simulink model "tesd"  (R2012b)
settings: Solver=ode45  StartTime=0.0  StopTime=25000  RelTol=1e-3
undefined symbols (not defined in the file or in its folder): pfb_coeff_gen_calc, sfp
undefined symbols (not defined in the file): SL, transtable
libraries: xbsIndex_r4 x5040, casper_library_misc x112, casper_library_delays x24, xps_library x14, maddogLibrary x4, simulink x2
(part 34 of 49)

== system tesd/FRD1/trIQ/tr/mem ==
  note: Undo data manipulation on way in and redo on way out for simulated data
  note: Undo address
      | manipulation for
      | simulated data
  In1 : Inport
  In2 : Inport  Port=2
  In3 : Inport  Port=3
  Disregard Subsystem : xbsIndex_r4/Disregard Subsystem  Tag=discardX  block_type=disregard
  calc_add : Subsystem  mask{data_width=32, addr_width=10, sample_rate=sample_rate}
      mask prompts: data_width "data width"; addr_width "address width"; sample_rate "sample rate"
  ram : xbsIndex_r4/Single Port RAM  depth=2^addr_width  initVector=init_vals  distributed_mem=Block RAM  write_mode=Read After Write  rst=off  init_reg=0  en=off  latency=1  dbl_ovrd=off  optimize=Area  block_type=spram
  sim_addr : xbsIndex_r4/Gateway In  gui_display_data_type=Fixed-point  arith_type=Unsigned  n_bits=addr_width  bin_pt=0  preci_type=Single  exp_width=8  frac_width=24  quantization=Truncate  overflow=Wrap  period=sample_rate  dbl_ovrd=off  timing_constraint=None  locs_specified=off  LOCs={}  UseAsADC=off  ADCChannel='1'  inherit_from_input=off  hdl_port=on  block_type=gatewayin
      settings: infoedit="Gateway in block.  Converts inputs of type Simulink integer, double and fixed point to  Xilinx fixed point type.<br><br>Hardware notes:  In hardware these blocks become top level input ports."  xl_area=[0, 0, 0, 0, 0, 0, 0]  sginterface={'Nallatech'=>{'xdspkit'=>{'non_memory_mapped_port'=>'sim_addr'}},'Xilinx'=>{'jtaghwcosim'=>{'non_memory_mapped_port'=>'sim_addr'},'xdspkit'=>{'non_memory_mapped_port'=>'sim_addr'}}}
  sim_data_in : xbsIndex_r4/Gateway In  gui_display_data_type=Fixed-point  arith_type=Unsigned  n_bits=32  bin_pt=0  preci_type=Single  exp_width=8  frac_width=24  quantization=Truncate  overflow=Wrap  period=sample_rate  dbl_ovrd=off  timing_constraint=None  locs_specified=off  LOCs={}  UseAsADC=off  ADCChannel='1'  inherit_from_input=off  hdl_port=on  block_type=gatewayin
      settings: xl_area=[0, 0, 0, 0, 0, 0, 0]  sginterface={'Nallatech'=>{'xdspkit'=>{'non_memory_mapped_port'=>'sim_data_in'}},'Xilinx'=>{'jtaghwcosim'=>{'non_memory_mapped_port'=>'sim_data_in'},'xdspkit'=>{'non_memory_mapped_port'=>'sim_data_in'}}}
  sim_data_out : xbsIndex_r4/Gateway Out  inherit_from_input=off  hdl_port=on  timing_constraint=None  locs_specified=off  LOCs={'B21','B22','A22','B23','B19','C19','A20','A21','A23','B24','A24','A25','E18','D18','C18','B18'}  UseAsDAC=off  DACChannel='1'  block_type=gatewayout
      settings: infoedit="Gateway out block.  Converts Xilinx fixed point inputs into ouputs of type Simulink integer, double, or fixed point.<P><P>Hardware notes:  In hardware these blocks become top level output ports or are discarded, depending on how they are configured."  xl_area=[0, 0, 0, 0, 0, 0, 0]  sginterface={'Nallatech'=>{'xdspkit'=>{'non_memory_mapped_port'=>'sim_data_out'}},'Xilinx'=>{'jtaghwcosim'=>{'non_memory_mapped_port'=>'sim_data_out'},'xdspkit'=>{'non_memory_mapped_port'=>'sim_data_out'}}}
  sim_munge_in : Subsystem  AncestorBlock=casper_library_flow_control/munge  mask(munge){divisions=1, div_size=32, order=[0], arith_type_out=Unsigned, bin_pt_out=0}
      mask prompts: divisions "Number of divisions"; div_size "Division size (bits)"; order "Division packing order"; arith_type_out "Output arithmetic type"; bin_pt_out "Output binary point"
      mask help: Splits an input bus into the specified number of divisions and then recombines them in the order specified (most significant division = 0,least = number divisions-1)
      mask init:
      | munge_init(gcb, ...
      |     'divisions', divisions, ...
      |     'div_size', div_size, ...
      |     'order', order, ...
      |     'arith_type_out', arith_type_out, ...
      |     'bin_pt_out', bin_pt_out);
      settings: AttributesFormatString=|
      | split:32
      | join:0
      | Unsigned [32,0]
      mask TypeOptions arith_type_out: Unsigned | Signed  (2's comp) | Floating-point
  sim_munge_out : Subsystem  AncestorBlock=casper_library_flow_control/munge  mask(munge){divisions=1, div_size=32, order=[0], arith_type_out=Unsigned, bin_pt_out=0}
      mask prompts: divisions "Number of divisions"; div_size "Division size (bits)"; order "Division packing order"; arith_type_out "Output arithmetic type"; bin_pt_out "Output binary point"
      mask help: Splits an input bus into the specified number of divisions and then recombines them in the order specified (most significant division = 0,least = number divisions-1)
      mask init:
      | munge_init(gcb, ...
      |     'divisions', divisions, ...
      |     'div_size', div_size, ...
      |     'order', order, ...
      |     'arith_type_out', arith_type_out, ...
      |     'bin_pt_out', bin_pt_out);
      settings: AttributesFormatString=|
      | split:32
      | join:0
      | Unsigned [32,0]
      mask TypeOptions arith_type_out: Unsigned | Signed  (2's comp) | Floating-point
  sim_we : xbsIndex_r4/Gateway In  gui_display_data_type=Fixed-point  arith_type=Boolean  n_bits=1  bin_pt=0  preci_type=Single  exp_width=8  frac_width=24  quantization=Truncate  overflow=Wrap  period=sample_rate  dbl_ovrd=off  timing_constraint=None  locs_specified=off  LOCs={}  UseAsADC=off  ADCChannel='1'  inherit_from_input=off  hdl_port=on  block_type=gatewayin
      settings: infoedit="Gateway in block.  Converts inputs of type Simulink integer, double and fixed point to  Xilinx fixed point type.<br><br>Hardware notes:  In hardware these blocks become top level input ports."  xl_area=[0, 0, 0, 0, 0, 0, 0]  sginterface={'Nallatech'=>{'xdspkit'=>{'non_memory_mapped_port'=>'sim_we'}},'Xilinx'=>{'jtaghwcosim'=>{'non_memory_mapped_port'=>'sim_we'},'xdspkit'=>{'non_memory_mapped_port'=>'sim_we'}}}
  Out1 : Outport
  wires:
  calc_add/1(out) -> ram/1
  sim_munge_out/1(dout) -> sim_data_out/1
  In1/1 -> sim_addr/1
  In2/1 -> sim_data_in/1
  sim_data_out/1 -> Out1/1
  In3/1 -> sim_we/1
  sim_addr/1 -> calc_add/1(in)
  sim_data_in/1 -> sim_munge_in/1(din)
  sim_we/1 -> ram/3
  ram/1 -> sim_munge_out/1(din)
  sim_munge_in/1(dout) -> ram/2

== system tesd/FRD1/trIQ/tr/munge_in ==
  din : Inport
  reinterpret_out : xbsIndex_r4/Reinterpret  force_arith_type=on  arith_type=Unsigned  force_bin_pt=on  bin_pt=0  block_type=reinterpret
  dout : Outport
  wires:
  reinterpret_out/1 -> dout/1
  din/1 -> reinterpret_out/1

== system tesd/FRD1/trIQ/tr/munge_out ==
  din : Inport
  reinterpret_out : xbsIndex_r4/Reinterpret  force_arith_type=on  arith_type=Unsigned  force_bin_pt=on  bin_pt=0  block_type=reinterpret
  dout : Outport
  wires:
  reinterpret_out/1 -> dout/1
  din/1 -> reinterpret_out/1

== system tesd/WindowAndFFT/FFT512_/FFT_DIT512_/Butterfly ==
  note: same delay as cmpkx mult
  ImInOne : Inport
  ReInOne : Inport  Port=2
  ImInTw : Inport  Port=3
  ReInTw : Inport  Port=4
  TwIm : Inport  Port=5
  TwRe : Inport  Port=6
  dvld : Inport  Port=7
  syncin : Inport  Port=8
  AddSub : xbsIndex_r4/AddSub  mode=Addition  use_carryin=off  use_carryout=off  en=off  latency=1  precision=Full  arith_type=Unsigned  n_bits=16  bin_pt=14  quantization=Truncate  overflow=Wrap  dbl_ovrd=off  use_behavioral_HDL=off  hw_selection=Fabric  pipelined=off  block_type=addsub
  AddSub1 : xbsIndex_r4/AddSub  mode=Addition  use_carryin=off  use_carryout=off  en=off  latency=1  precision=Full  arith_type=Unsigned  n_bits=16  bin_pt=14  quantization=Truncate  overflow=Wrap  dbl_ovrd=off  use_behavioral_HDL=off  hw_selection=Fabric  pipelined=off  block_type=addsub
  "Complex Multiplier 5.0 " : xbsIndex_r4/Complex Multiplier 5.0   hasatlast=on  hasatuser=off  atuserwidth=1  hasbtlast=off  hasbtuser=off  btuserwidth=1  multtype=Use_Mults  optimizegoal=Resources  flowcontrol=NonBlocking  outputwidth=33  roundmode=Truncate  hasctrltlast=off  hasctrltuser=off  ctrltuserwidth=1  outtlastbehv=Pass_A_TLAST  latencyconfig=Automatic  minimumlatency=37  aclken=off  aresetn=off  trim_axipin_name=on  aportwidth=63  bportwidth=63  ip_name=Complex Multiplier  ip_version=5.0  dsptool_ready=true  ipcore_usecache=true  ipcore_useipmodelcache=true  ipcore_verbose=false  ipcore_latency_parameter='minimumlatency'  wrapper_available=true  port_translation_map={ 'aclken' => 'en', 'aresetn' => 'rst'}  structural_sim=false  block_type=cmpy_v5_0
  Complex to Magnitude-Angle{,1..5} (6 alike) : ComplexToMagnitudeAngle
  Convert{,1..7} (8 alike) : xbsIndex_r4/Convert  gui_display_data_type=Fixed-point  arith_type="Signed  (2's comp)"  n_bits=16  bin_pt=14  float_type=Single  exp_bits=8  fraction_bits=24  quantization=Truncate  overflow=Wrap  en=off  latency=0  dbl_ovrd=off  pipeline=off  block_type=convert
  Delay : xbsIndex_r4/Delay  rst=off  infoeditControl=Selection of Reset will increase slice count due to use of real FFs and instead of SRLs  en=off  latency=6  dbl_ovrd=off  reg_retiming=off  block_type=delay
  Delay1 : xbsIndex_r4/Delay  rst=off  infoeditControl=Selection of Reset will increase slice count due to use of real FFs and instead of SRLs  en=off  latency=6  dbl_ovrd=off  reg_retiming=off  block_type=delay
  Delay2 : xbsIndex_r4/Delay  rst=off  infoeditControl=Selection of Reset will increase slice count due to use of real FFs and instead of SRLs  en=off  latency=1  dbl_ovrd=off  reg_retiming=off  block_type=delay
  Delay3 : xbsIndex_r4/Delay  rst=off  infoeditControl=Selection of Reset will increase slice count due to use of real FFs and instead of SRLs  en=off  latency=1  dbl_ovrd=off  reg_retiming=off  block_type=delay
  Gateway Out{1..14} (14 alike) : xbsIndex_r4/Gateway Out  inherit_from_input=off  hdl_port=on  timing_constraint=None  locs_specified=off  LOCs={}  UseAsDAC=off  DACChannel='1'  block_type=gatewayout
  Real-Imag to Complex{,1..5} (6 alike) : RealImagToComplex
  buttscope : Scope  NumInputPorts=6
      settings: YMin=-5~-5~-5~-5~-5~-5  YMax=5~5~5~5~5~5  SaveName=ScopeData4
  buttscope1 : Scope  NumInputPorts=8
      settings: YMin=-5~-5~-5~-5~-5~-5~-5~-5  YMax=5~5~5~5~5~5~5~5  SaveName=ScopeData6
  Imut : Outport
  ReOut : Outport  Port=2
  dvldout : Outport  Port=3
  syncout : Outport  Port=4
  wires:
  ReInOne/1 -> Convert7/1
  ImInOne/1 -> Convert6/1
  AddSub/1 -> Gateway Out6/1, Imut/1
  AddSub1/1 -> Gateway Out2/1, ReOut/1
  ImInTw/1 -> Convert3/1
  ReInTw/1 -> Convert2/1
  Delay/1 -> Gateway Out7/1, AddSub/1
  Delay1/1 -> Gateway Out3/1, AddSub1/1
  TwIm/1 -> Convert4/1
  TwRe/1 -> Convert5/1
  dvld/1 -> "Complex Multiplier 5.0 "/5, "Complex Multiplier 5.0 "/1
  Convert6/1 -> Delay/1
  Convert7/1 -> Delay1/1
  Convert3/1 -> "Complex Multiplier 5.0 "/3, Gateway Out11/1
  Convert2/1 -> "Complex Multiplier 5.0 "/4, Gateway Out12/1
  Convert4/1 -> "Complex Multiplier 5.0 "/6, Gateway Out5/1
  Convert5/1 -> "Complex Multiplier 5.0 "/7, Gateway Out8/1
  Convert1/1 -> Gateway Out10/1, Gateway Out4/1, AddSub1/2
  syncin/1 -> Gateway Out14/1, "Complex Multiplier 5.0 "/2
  "Complex Multiplier 5.0 "/4 -> Convert1/1
  "Complex Multiplier 5.0 "/3 -> Convert/1
  "Complex Multiplier 5.0 "/1 -> Delay2/1
  "Complex Multiplier 5.0 "/2 -> Gateway Out13/1, Delay3/1
  Convert/1 -> Gateway Out9/1, Gateway Out1/1, AddSub/2
  Delay2/1 -> dvldout/1
  Delay3/1 -> syncout/1
  Real-Imag to Complex/1 -> Complex to Magnitude-Angle/1
  Real-Imag to Complex1/1 -> Complex to Magnitude-Angle1/1
  Real-Imag to Complex2/1 -> Complex to Magnitude-Angle2/1
  Complex to Magnitude-Angle/1 -> buttscope1/1
  Complex to Magnitude-Angle/2 -> buttscope1/2
  Complex to Magnitude-Angle1/1 -> buttscope1/3
  Complex to Magnitude-Angle1/2 -> buttscope1/4
  Complex to Magnitude-Angle2/1 -> buttscope1/5
  Complex to Magnitude-Angle2/2 -> buttscope1/6
  Gateway Out11/1 -> Real-Imag to Complex/2
  Gateway Out12/1 -> Real-Imag to Complex/1
  Gateway Out5/1 -> Real-Imag to Complex1/2
  Gateway Out8/1 -> Real-Imag to Complex1/1
  Gateway Out9/1 -> Real-Imag to Complex2/2
  Gateway Out10/1 -> Real-Imag to Complex2/1
  Gateway Out13/1 -> buttscope1/7
  Gateway Out14/1 -> buttscope1/8
  Real-Imag to Complex3/1 -> Complex to Magnitude-Angle3/1
  Real-Imag to Complex4/1 -> Complex to Magnitude-Angle4/1
  Real-Imag to Complex5/1 -> Complex to Magnitude-Angle5/1
  Gateway Out7/1 -> Real-Imag to Complex3/2
  Gateway Out3/1 -> Real-Imag to Complex3/1
  Complex to Magnitude-Angle3/1 -> buttscope/1
  Complex to Magnitude-Angle3/2 -> buttscope/2
  Gateway Out1/1 -> Real-Imag to Complex4/2
  Gateway Out4/1 -> Real-Imag to Complex4/1
  Complex to Magnitude-Angle4/1 -> buttscope/3
  Complex to Magnitude-Angle4/2 -> buttscope/4
  Gateway Out6/1 -> Real-Imag to Complex5/2
  Gateway Out2/1 -> Real-Imag to Complex5/1
  Complex to Magnitude-Angle5/1 -> buttscope/5
  Complex to Magnitude-Angle5/2 -> buttscope/6

== system tesd/WindowAndFFT/FFT512_/FFT_DIT512_/Butterfly1 ==
  note: same delay as cmpkx mult
  ImInOne : Inport
  ReInOne : Inport  Port=2
  ImInTw : Inport  Port=3
  ReInTw : Inport  Port=4
  TwIm : Inport  Port=5
  TwRe : Inport  Port=6
  dvld : Inport  Port=7
  syncin : Inport  Port=8
  AddSub : xbsIndex_r4/AddSub  mode=Addition  use_carryin=off  use_carryout=off  en=off  latency=1  precision=Full  arith_type=Unsigned  n_bits=16  bin_pt=14  quantization=Truncate  overflow=Wrap  dbl_ovrd=off  use_behavioral_HDL=off  hw_selection=Fabric  pipelined=off  block_type=addsub
  AddSub1 : xbsIndex_r4/AddSub  mode=Addition  use_carryin=off  use_carryout=off  en=off  latency=1  precision=Full  arith_type=Unsigned  n_bits=16  bin_pt=14  quantization=Truncate  overflow=Wrap  dbl_ovrd=off  use_behavioral_HDL=off  hw_selection=Fabric  pipelined=off  block_type=addsub
  "Complex Multiplier 5.0 " : xbsIndex_r4/Complex Multiplier 5.0   hasatlast=on  hasatuser=off  atuserwidth=1  hasbtlast=off  hasbtuser=off  btuserwidth=1  multtype=Use_Mults  optimizegoal=Resources  flowcontrol=NonBlocking  outputwidth=33  roundmode=Truncate  hasctrltlast=off  hasctrltuser=off  ctrltuserwidth=1  outtlastbehv=Pass_A_TLAST  latencyconfig=Automatic  minimumlatency=37  aclken=off  aresetn=off  trim_axipin_name=on  aportwidth=63  bportwidth=63  ip_name=Complex Multiplier  ip_version=5.0  dsptool_ready=true  ipcore_usecache=true  ipcore_useipmodelcache=true  ipcore_verbose=false  ipcore_latency_parameter='minimumlatency'  wrapper_available=true  port_translation_map={ 'aclken' => 'en', 'aresetn' => 'rst'}  structural_sim=false  block_type=cmpy_v5_0
  Complex to Magnitude-Angle{,1..5} (6 alike) : ComplexToMagnitudeAngle
  Convert{,1..7} (8 alike) : xbsIndex_r4/Convert  gui_display_data_type=Fixed-point  arith_type="Signed  (2's comp)"  n_bits=16  bin_pt=14  float_type=Single  exp_bits=8  fraction_bits=24  quantization=Truncate  overflow=Wrap  en=off  latency=0  dbl_ovrd=off  pipeline=off  block_type=convert
  Delay : xbsIndex_r4/Delay  rst=off  infoeditControl=Selection of Reset will increase slice count due to use of real FFs and instead of SRLs  en=off  latency=6  dbl_ovrd=off  reg_retiming=off  block_type=delay
  Delay1 : xbsIndex_r4/Delay  rst=off  infoeditControl=Selection of Reset will increase slice count due to use of real FFs and instead of SRLs  en=off  latency=6  dbl_ovrd=off  reg_retiming=off  block_type=delay
  Delay2 : xbsIndex_r4/Delay  rst=off  infoeditControl=Selection of Reset will increase slice count due to use of real FFs and instead of SRLs  en=off  latency=1  dbl_ovrd=off  reg_retiming=off  block_type=delay
  Delay3 : xbsIndex_r4/Delay  rst=off  infoeditControl=Selection of Reset will increase slice count due to use of real FFs and instead of SRLs  en=off  latency=1  dbl_ovrd=off  reg_retiming=off  block_type=delay
  Gateway Out{1..14} (14 alike) : xbsIndex_r4/Gateway Out  inherit_from_input=off  hdl_port=on  timing_constraint=None  locs_specified=off  LOCs={}  UseAsDAC=off  DACChannel='1'  block_type=gatewayout
  Real-Imag to Complex{,1..5} (6 alike) : RealImagToComplex
  buttscope : Scope  NumInputPorts=6
      settings: YMin=-5~-5~-5~-5~-5~-5  YMax=5~5~5~5~5~5  SaveName=ScopeData4
  buttscope1 : Scope  NumInputPorts=8
      settings: YMin=-5~-5~-5~-5~-5~-5~-5~-5  YMax=5~5~5~5~5~5~5~5  SaveName=ScopeData6
  Imut : Outport
  ReOut : Outport  Port=2
  dvldout : Outport  Port=3
  syncout : Outport  Port=4
  wires:
  ReInOne/1 -> Convert7/1
  ImInOne/1 -> Convert6/1
  AddSub/1 -> Gateway Out6/1, Imut/1
  AddSub1/1 -> Gateway Out2/1, ReOut/1
  ImInTw/1 -> Convert3/1
  ReInTw/1 -> Convert2/1
  Delay/1 -> Gateway Out7/1, AddSub/1
  Delay1/1 -> Gateway Out3/1, AddSub1/1
  TwIm/1 -> Convert4/1
  TwRe/1 -> Convert5/1
  dvld/1 -> "Complex Multiplier 5.0 "/5, "Complex Multiplier 5.0 "/1
  Convert6/1 -> Delay/1
  Convert7/1 -> Delay1/1
  Convert3/1 -> "Complex Multiplier 5.0 "/3, Gateway Out11/1
  Convert2/1 -> "Complex Multiplier 5.0 "/4, Gateway Out12/1
  Convert4/1 -> "Complex Multiplier 5.0 "/6, Gateway Out5/1
  Convert5/1 -> "Complex Multiplier 5.0 "/7, Gateway Out8/1
  Convert1/1 -> Gateway Out10/1, Gateway Out4/1, AddSub1/2
  syncin/1 -> Gateway Out14/1, "Complex Multiplier 5.0 "/2
  "Complex Multiplier 5.0 "/4 -> Convert1/1
  "Complex Multiplier 5.0 "/3 -> Convert/1
  "Complex Multiplier 5.0 "/1 -> Delay2/1
  "Complex Multiplier 5.0 "/2 -> Gateway Out13/1, Delay3/1
  Convert/1 -> Gateway Out9/1, Gateway Out1/1, AddSub/2
  Delay2/1 -> dvldout/1
  Delay3/1 -> syncout/1
  Real-Imag to Complex/1 -> Complex to Magnitude-Angle/1
  Real-Imag to Complex1/1 -> Complex to Magnitude-Angle1/1
  Real-Imag to Complex2/1 -> Complex to Magnitude-Angle2/1
  Complex to Magnitude-Angle/1 -> buttscope1/1
  Complex to Magnitude-Angle/2 -> buttscope1/2
  Complex to Magnitude-Angle1/1 -> buttscope1/3
  Complex to Magnitude-Angle1/2 -> buttscope1/4
  Complex to Magnitude-Angle2/1 -> buttscope1/5
  Complex to Magnitude-Angle2/2 -> buttscope1/6
  Gateway Out11/1 -> Real-Imag to Complex/2
  Gateway Out12/1 -> Real-Imag to Complex/1
  Gateway Out5/1 -> Real-Imag to Complex1/2
  Gateway Out8/1 -> Real-Imag to Complex1/1
  Gateway Out9/1 -> Real-Imag to Complex2/2
  Gateway Out10/1 -> Real-Imag to Complex2/1
  Gateway Out13/1 -> buttscope1/7
  Gateway Out14/1 -> buttscope1/8
  Real-Imag to Complex3/1 -> Complex to Magnitude-Angle3/1
  Real-Imag to Complex4/1 -> Complex to Magnitude-Angle4/1
  Real-Imag to Complex5/1 -> Complex to Magnitude-Angle5/1
  Gateway Out7/1 -> Real-Imag to Complex3/2
  Gateway Out3/1 -> Real-Imag to Complex3/1
  Complex to Magnitude-Angle3/1 -> buttscope/1
  Complex to Magnitude-Angle3/2 -> buttscope/2
  Gateway Out1/1 -> Real-Imag to Complex4/2
  Gateway Out4/1 -> Real-Imag to Complex4/1
  Complex to Magnitude-Angle4/1 -> buttscope/3
  Complex to Magnitude-Angle4/2 -> buttscope/4
  Gateway Out6/1 -> Real-Imag to Complex5/2
  Gateway Out2/1 -> Real-Imag to Complex5/1
  Complex to Magnitude-Angle5/1 -> buttscope/5
  Complex to Magnitude-Angle5/2 -> buttscope/6

== system tesd/WindowAndFFT/FFT512_/FFT_DIT512_/Butterfly2 ==
  note: same delay as cmpkx mult
  ImInOne : Inport
  ReInOne : Inport  Port=2
  ImInTw : Inport  Port=3
  ReInTw : Inport  Port=4
  TwIm : Inport  Port=5
  TwRe : Inport  Port=6
  dvld : Inport  Port=7
  syncin : Inport  Port=8
  AddSub : xbsIndex_r4/AddSub  mode=Addition  use_carryin=off  use_carryout=off  en=off  latency=1  precision=Full  arith_type=Unsigned  n_bits=16  bin_pt=14  quantization=Truncate  overflow=Wrap  dbl_ovrd=off  use_behavioral_HDL=off  hw_selection=Fabric  pipelined=off  block_type=addsub
  AddSub1 : xbsIndex_r4/AddSub  mode=Addition  use_carryin=off  use_carryout=off  en=off  latency=1  precision=Full  arith_type=Unsigned  n_bits=16  bin_pt=14  quantization=Truncate  overflow=Wrap  dbl_ovrd=off  use_behavioral_HDL=off  hw_selection=Fabric  pipelined=off  block_type=addsub
  "Complex Multiplier 5.0 " : xbsIndex_r4/Complex Multiplier 5.0   hasatlast=on  hasatuser=off  atuserwidth=1  hasbtlast=off  hasbtuser=off  btuserwidth=1  multtype=Use_Mults  optimizegoal=Resources  flowcontrol=NonBlocking  outputwidth=33  roundmode=Truncate  hasctrltlast=off  hasctrltuser=off  ctrltuserwidth=1  outtlastbehv=Pass_A_TLAST  latencyconfig=Automatic  minimumlatency=37  aclken=off  aresetn=off  trim_axipin_name=on  aportwidth=63  bportwidth=63  ip_name=Complex Multiplier  ip_version=5.0  dsptool_ready=true  ipcore_usecache=true  ipcore_useipmodelcache=true  ipcore_verbose=false  ipcore_latency_parameter='minimumlatency'  wrapper_available=true  port_translation_map={ 'aclken' => 'en', 'aresetn' => 'rst'}  structural_sim=false  block_type=cmpy_v5_0
  Complex to Magnitude-Angle{,1..5} (6 alike) : ComplexToMagnitudeAngle
  Convert{,1..7} (8 alike) : xbsIndex_r4/Convert  gui_display_data_type=Fixed-point  arith_type="Signed  (2's comp)"  n_bits=16  bin_pt=14  float_type=Single  exp_bits=8  fraction_bits=24  quantization=Truncate  overflow=Wrap  en=off  latency=0  dbl_ovrd=off  pipeline=off  block_type=convert
  Delay : xbsIndex_r4/Delay  rst=off  infoeditControl=Selection of Reset will increase slice count due to use of real FFs and instead of SRLs  en=off  latency=6  dbl_ovrd=off  reg_retiming=off  block_type=delay
  Delay1 : xbsIndex_r4/Delay  rst=off  infoeditControl=Selection of Reset will increase slice count due to use of real FFs and instead of SRLs  en=off  latency=6  dbl_ovrd=off  reg_retiming=off  block_type=delay
  Delay2 : xbsIndex_r4/Delay  rst=off  infoeditControl=Selection of Reset will increase slice count due to use of real FFs and instead of SRLs  en=off  latency=1  dbl_ovrd=off  reg_retiming=off  block_type=delay
  Delay3 : xbsIndex_r4/Delay  rst=off  infoeditControl=Selection of Reset will increase slice count due to use of real FFs and instead of SRLs  en=off  latency=1  dbl_ovrd=off  reg_retiming=off  block_type=delay
  Gateway Out{1..14} (14 alike) : xbsIndex_r4/Gateway Out  inherit_from_input=off  hdl_port=on  timing_constraint=None  locs_specified=off  LOCs={}  UseAsDAC=off  DACChannel='1'  block_type=gatewayout
  Real-Imag to Complex{,1..5} (6 alike) : RealImagToComplex
  buttscope : Scope  NumInputPorts=6
      settings: YMin=-5~-5~-5~-5~-5~-5  YMax=5~5~5~5~5~5  SaveName=ScopeData4
  buttscope1 : Scope  NumInputPorts=8
      settings: YMin=-5~-5~-5~-5~-5~-5~-5~-5  YMax=5~5~5~5~5~5~5~5  SaveName=ScopeData6
  Imut : Outport
  ReOut : Outport  Port=2
  dvldout : Outport  Port=3
  syncout : Outport  Port=4
  wires:
  ReInOne/1 -> Convert7/1
  ImInOne/1 -> Convert6/1
  AddSub/1 -> Gateway Out6/1, Imut/1
  AddSub1/1 -> Gateway Out2/1, ReOut/1
  ImInTw/1 -> Convert3/1
  ReInTw/1 -> Convert2/1
  Delay/1 -> Gateway Out7/1, AddSub/1
  Delay1/1 -> Gateway Out3/1, AddSub1/1
  TwIm/1 -> Convert4/1
  TwRe/1 -> Convert5/1
  dvld/1 -> "Complex Multiplier 5.0 "/5, "Complex Multiplier 5.0 "/1
  Convert6/1 -> Delay/1
  Convert7/1 -> Delay1/1
  Convert3/1 -> "Complex Multiplier 5.0 "/3, Gateway Out11/1
  Convert2/1 -> "Complex Multiplier 5.0 "/4, Gateway Out12/1
  Convert4/1 -> "Complex Multiplier 5.0 "/6, Gateway Out5/1
  Convert5/1 -> "Complex Multiplier 5.0 "/7, Gateway Out8/1
  Convert1/1 -> Gateway Out10/1, Gateway Out4/1, AddSub1/2
  syncin/1 -> Gateway Out14/1, "Complex Multiplier 5.0 "/2
  "Complex Multiplier 5.0 "/4 -> Convert1/1
  "Complex Multiplier 5.0 "/3 -> Convert/1
  "Complex Multiplier 5.0 "/1 -> Delay2/1
  "Complex Multiplier 5.0 "/2 -> Gateway Out13/1, Delay3/1
  Convert/1 -> Gateway Out9/1, Gateway Out1/1, AddSub/2
  Delay2/1 -> dvldout/1
  Delay3/1 -> syncout/1
  Real-Imag to Complex/1 -> Complex to Magnitude-Angle/1
  Real-Imag to Complex1/1 -> Complex to Magnitude-Angle1/1
  Real-Imag to Complex2/1 -> Complex to Magnitude-Angle2/1
  Complex to Magnitude-Angle/1 -> buttscope1/1
  Complex to Magnitude-Angle/2 -> buttscope1/2
  Complex to Magnitude-Angle1/1 -> buttscope1/3
  Complex to Magnitude-Angle1/2 -> buttscope1/4
  Complex to Magnitude-Angle2/1 -> buttscope1/5
  Complex to Magnitude-Angle2/2 -> buttscope1/6
  Gateway Out11/1 -> Real-Imag to Complex/2
  Gateway Out12/1 -> Real-Imag to Complex/1
  Gateway Out5/1 -> Real-Imag to Complex1/2
  Gateway Out8/1 -> Real-Imag to Complex1/1
  Gateway Out9/1 -> Real-Imag to Complex2/2
  Gateway Out10/1 -> Real-Imag to Complex2/1
  Gateway Out13/1 -> buttscope1/7
  Gateway Out14/1 -> buttscope1/8
  Real-Imag to Complex3/1 -> Complex to Magnitude-Angle3/1
  Real-Imag to Complex4/1 -> Complex to Magnitude-Angle4/1
  Real-Imag to Complex5/1 -> Complex to Magnitude-Angle5/1
  Gateway Out7/1 -> Real-Imag to Complex3/2
  Gateway Out3/1 -> Real-Imag to Complex3/1
  Complex to Magnitude-Angle3/1 -> buttscope/1
  Complex to Magnitude-Angle3/2 -> buttscope/2
  Gateway Out1/1 -> Real-Imag to Complex4/2
  Gateway Out4/1 -> Real-Imag to Complex4/1
  Complex to Magnitude-Angle4/1 -> buttscope/3
  Complex to Magnitude-Angle4/2 -> buttscope/4
  Gateway Out6/1 -> Real-Imag to Complex5/2
  Gateway Out2/1 -> Real-Imag to Complex5/1
  Complex to Magnitude-Angle5/1 -> buttscope/5
  Complex to Magnitude-Angle5/2 -> buttscope/6

== system tesd/WindowAndFFT/FFT512_/FFT_DIT512_/Butterfly3 ==
  note: same delay as cmpkx mult
  ImInOne : Inport
  ReInOne : Inport  Port=2
  ImInTw : Inport  Port=3
  ReInTw : Inport  Port=4
  TwIm : Inport  Port=5
  TwRe : Inport  Port=6
  dvld : Inport  Port=7
  syncin : Inport  Port=8
  AddSub : xbsIndex_r4/AddSub  mode=Addition  use_carryin=off  use_carryout=off  en=off  latency=1  precision=Full  arith_type=Unsigned  n_bits=16  bin_pt=14  quantization=Truncate  overflow=Wrap  dbl_ovrd=off  use_behavioral_HDL=off  hw_selection=Fabric  pipelined=off  block_type=addsub
  AddSub1 : xbsIndex_r4/AddSub  mode=Addition  use_carryin=off  use_carryout=off  en=off  latency=1  precision=Full  arith_type=Unsigned  n_bits=16  bin_pt=14  quantization=Truncate  overflow=Wrap  dbl_ovrd=off  use_behavioral_HDL=off  hw_selection=Fabric  pipelined=off  block_type=addsub
  "Complex Multiplier 5.0 " : xbsIndex_r4/Complex Multiplier 5.0   hasatlast=on  hasatuser=off  atuserwidth=1  hasbtlast=off  hasbtuser=off  btuserwidth=1  multtype=Use_Mults  optimizegoal=Resources  flowcontrol=NonBlocking  outputwidth=33  roundmode=Truncate  hasctrltlast=off  hasctrltuser=off  ctrltuserwidth=1  outtlastbehv=Pass_A_TLAST  latencyconfig=Automatic  minimumlatency=37  aclken=off  aresetn=off  trim_axipin_name=on  aportwidth=63  bportwidth=63  ip_name=Complex Multiplier  ip_version=5.0  dsptool_ready=true  ipcore_usecache=true  ipcore_useipmodelcache=true  ipcore_verbose=false  ipcore_latency_parameter='minimumlatency'  wrapper_available=true  port_translation_map={ 'aclken' => 'en', 'aresetn' => 'rst'}  structural_sim=false  block_type=cmpy_v5_0
  Complex to Magnitude-Angle{,1..5} (6 alike) : ComplexToMagnitudeAngle
  Convert{,1..7} (8 alike) : xbsIndex_r4/Convert  gui_display_data_type=Fixed-point  arith_type="Signed  (2's comp)"  n_bits=16  bin_pt=14  float_type=Single  exp_bits=8  fraction_bits=24  quantization=Truncate  overflow=Wrap  en=off  latency=0  dbl_ovrd=off  pipeline=off  block_type=convert
  Delay : xbsIndex_r4/Delay  rst=off  infoeditControl=Selection of Reset will increase slice count due to use of real FFs and instead of SRLs  en=off  latency=6  dbl_ovrd=off  reg_retiming=off  block_type=delay
  Delay1 : xbsIndex_r4/Delay  rst=off  infoeditControl=Selection of Reset will increase slice count due to use of real FFs and instead of SRLs  en=off  latency=6  dbl_ovrd=off  reg_retiming=off  block_type=delay
  Delay2 : xbsIndex_r4/Delay  rst=off  infoeditControl=Selection of Reset will increase slice count due to use of real FFs and instead of SRLs  en=off  latency=1  dbl_ovrd=off  reg_retiming=off  block_type=delay
  Delay3 : xbsIndex_r4/Delay  rst=off  infoeditControl=Selection of Reset will increase slice count due to use of real FFs and instead of SRLs  en=off  latency=1  dbl_ovrd=off  reg_retiming=off  block_type=delay
  Gateway Out{1..14} (14 alike) : xbsIndex_r4/Gateway Out  inherit_from_input=off  hdl_port=on  timing_constraint=None  locs_specified=off  LOCs={}  UseAsDAC=off  DACChannel='1'  block_type=gatewayout
  Real-Imag to Complex{,1..5} (6 alike) : RealImagToComplex
  buttscope : Scope  NumInputPorts=6
      settings: YMin=-5~-5~-5~-5~-5~-5  YMax=5~5~5~5~5~5  SaveName=ScopeData4
  buttscope1 : Scope  NumInputPorts=8
      settings: YMin=-5~-5~-5~-5~-5~-5~-5~-5  YMax=5~5~5~5~5~5~5~5  SaveName=ScopeData6
  Imut : Outport
  ReOut : Outport  Port=2
  dvldout : Outport  Port=3
  syncout : Outport  Port=4
  wires:
  ReInOne/1 -> Convert7/1
  ImInOne/1 -> Convert6/1
  AddSub/1 -> Gateway Out6/1, Imut/1
  AddSub1/1 -> Gateway Out2/1, ReOut/1
  ImInTw/1 -> Convert3/1
  ReInTw/1 -> Convert2/1
  Delay/1 -> Gateway Out7/1, AddSub/1
  Delay1/1 -> Gateway Out3/1, AddSub1/1
  TwIm/1 -> Convert4/1
  TwRe/1 -> Convert5/1
  dvld/1 -> "Complex Multiplier 5.0 "/5, "Complex Multiplier 5.0 "/1
  Convert6/1 -> Delay/1
  Convert7/1 -> Delay1/1
  Convert3/1 -> "Complex Multiplier 5.0 "/3, Gateway Out11/1
  Convert2/1 -> "Complex Multiplier 5.0 "/4, Gateway Out12/1
  Convert4/1 -> "Complex Multiplier 5.0 "/6, Gateway Out5/1
  Convert5/1 -> "Complex Multiplier 5.0 "/7, Gateway Out8/1
  Convert1/1 -> Gateway Out10/1, Gateway Out4/1, AddSub1/2
  syncin/1 -> Gateway Out14/1, "Complex Multiplier 5.0 "/2
  "Complex Multiplier 5.0 "/4 -> Convert1/1
  "Complex Multiplier 5.0 "/3 -> Convert/1
  "Complex Multiplier 5.0 "/1 -> Delay2/1
  "Complex Multiplier 5.0 "/2 -> Gateway Out13/1, Delay3/1
  Convert/1 -> Gateway Out9/1, Gateway Out1/1, AddSub/2
  Delay2/1 -> dvldout/1
  Delay3/1 -> syncout/1
  Real-Imag to Complex/1 -> Complex to Magnitude-Angle/1
  Real-Imag to Complex1/1 -> Complex to Magnitude-Angle1/1
  Real-Imag to Complex2/1 -> Complex to Magnitude-Angle2/1
  Complex to Magnitude-Angle/1 -> buttscope1/1
  Complex to Magnitude-Angle/2 -> buttscope1/2
  Complex to Magnitude-Angle1/1 -> buttscope1/3
  Complex to Magnitude-Angle1/2 -> buttscope1/4
  Complex to Magnitude-Angle2/1 -> buttscope1/5
  Complex to Magnitude-Angle2/2 -> buttscope1/6
  Gateway Out11/1 -> Real-Imag to Complex/2
  Gateway Out12/1 -> Real-Imag to Complex/1
  Gateway Out5/1 -> Real-Imag to Complex1/2
  Gateway Out8/1 -> Real-Imag to Complex1/1
  Gateway Out9/1 -> Real-Imag to Complex2/2
  Gateway Out10/1 -> Real-Imag to Complex2/1
  Gateway Out13/1 -> buttscope1/7
  Gateway Out14/1 -> buttscope1/8
  Real-Imag to Complex3/1 -> Complex to Magnitude-Angle3/1
  Real-Imag to Complex4/1 -> Complex to Magnitude-Angle4/1
  Real-Imag to Complex5/1 -> Complex to Magnitude-Angle5/1
  Gateway Out7/1 -> Real-Imag to Complex3/2
  Gateway Out3/1 -> Real-Imag to Complex3/1
  Complex to Magnitude-Angle3/1 -> buttscope/1
  Complex to Magnitude-Angle3/2 -> buttscope/2
  Gateway Out1/1 -> Real-Imag to Complex4/2
  Gateway Out4/1 -> Real-Imag to Complex4/1
  Complex to Magnitude-Angle4/1 -> buttscope/3
  Complex to Magnitude-Angle4/2 -> buttscope/4
  Gateway Out6/1 -> Real-Imag to Complex5/2
  Gateway Out2/1 -> Real-Imag to Complex5/1
  Complex to Magnitude-Angle5/1 -> buttscope/5
  Complex to Magnitude-Angle5/2 -> buttscope/6

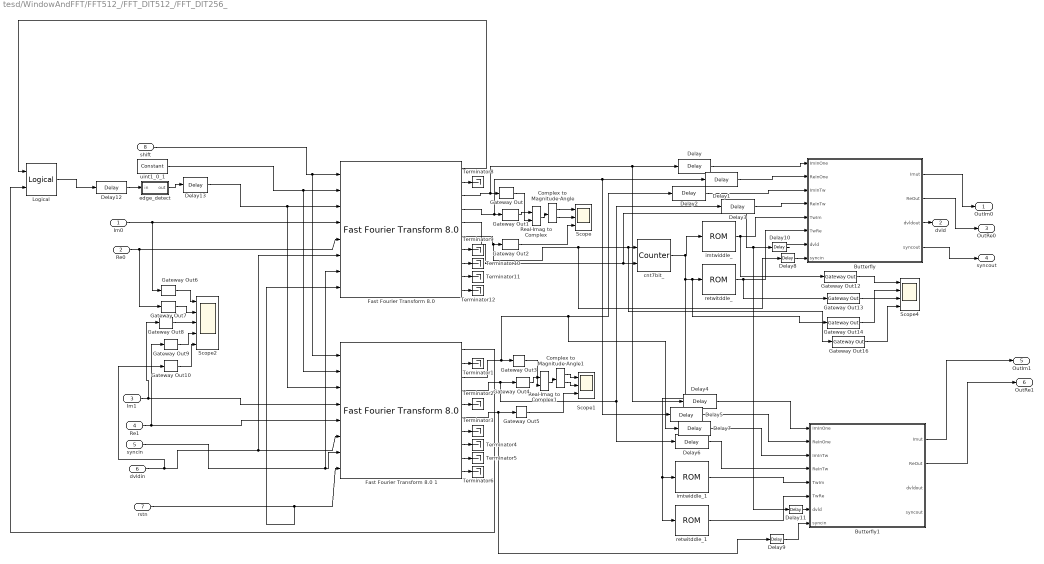
== system tesd/WindowAndFFT/FFT512_/FFT_DIT512_/FFT_DIT256_ ==
  Im0 : Inport
  Re0 : Inport  Port=2
  Im1 : Inport  Port=3
  Re1 : Inport  Port=4
  syncin : Inport  Port=5
  dvldin : Inport  Port=6
  rstn : Inport  Port=7
  shift : Inport  Port=8
  Butterfly : Subsystem
  Butterfly1 : Subsystem
  Complex to Magnitude-Angle : ComplexToMagnitudeAngle
  Complex to Magnitude-Angle1 : ComplexToMagnitudeAngle
  Delay{,1..12} (13 alike) : xbsIndex_r4/Delay  rst=off  infoeditControl=Selection of Reset will increase slice count due to use of real FFs and instead of SRLs  en=off  latency=1  dbl_ovrd=off  reg_retiming=off  block_type=delay
  Delay13 : xbsIndex_r4/Delay  rst=off  infoeditControl=Selection of Reset will increase slice count due to use of real FFs and instead of SRLs  en=off  latency=4  dbl_ovrd=off  reg_retiming=off  block_type=delay
  "Fast Fourier Transform 8.0 " : xbsIndex_r4/Fast Fourier Transform 8.0   transform_length=128  target_clock_frequency=128  target_data_throughput=50  implementation_options=pipelined_streaming_io  run_time_configurable_transform_length=off  phase_factor_width=16  scaling_options=scaled  rounding_modes=truncation  aclken=off  aresetn=on  cyclic_prefix_insertion=off  output_ordering=natural_order  throttle_scheme=realtime  xk_index=off  ovflo=off  trim_axipin_name=on  memory_options_data=block_ram  memory_options_phase_factors=block_ram  number_of_stages_using_block_ram_for_data_and_phase_factors=1  memory_options_reorder=block_ram  memory_options_hybrid=off  complex_mult_type=use_mults_resources  butterfly_type=use_luts  channels=1  input_ordering=natural_order  input_width=16  ip_name=Fast Fourier Transform  ip_version=8.0  dsptool_ready=true  ipcore_usecache=true  ipcore_useipmodelcache=true  wrapper_available=true  port_translation_map={ 'aclken' => 'en', 'aresetn' => 'rst'}  block_type=xfft_v8_0
  Fast Fourier Transform 8.0 1 : xbsIndex_r4/Fast Fourier Transform 8.0   transform_length=128  target_clock_frequency=128  target_data_throughput=50  implementation_options=pipelined_streaming_io  run_time_configurable_transform_length=off  phase_factor_width=16  scaling_options=scaled  rounding_modes=truncation  aclken=off  aresetn=on  cyclic_prefix_insertion=off  output_ordering=natural_order  throttle_scheme=realtime  xk_index=off  ovflo=off  trim_axipin_name=on  memory_options_data=block_ram  memory_options_phase_factors=block_ram  number_of_stages_using_block_ram_for_data_and_phase_factors=1  memory_options_reorder=block_ram  memory_options_hybrid=off  complex_mult_type=use_mults_resources  butterfly_type=use_luts  channels=1  input_ordering=natural_order  input_width=16  ip_name=Fast Fourier Transform  ip_version=8.0  dsptool_ready=true  ipcore_usecache=true  ipcore_useipmodelcache=true  wrapper_available=true  port_translation_map={ 'aclken' => 'en', 'aresetn' => 'rst'}  block_type=xfft_v8_0
  Gateway Out{,1..10,12..14,16} (15 alike) : xbsIndex_r4/Gateway Out  inherit_from_input=off  hdl_port=on  timing_constraint=None  locs_specified=off  LOCs={}  UseAsDAC=off  DACChannel='1'  block_type=gatewayout
  Logical : xbsIndex_r4/Logical  logical_function=AND  inputs=2  en=off  latency=0  precision=Full  arith_type=Unsigned  n_bits=16  bin_pt=0  align_bp=on  dbl_ovrd=off  block_type=logical
  Real-Imag to Complex : RealImagToComplex
  Real-Imag to Complex1 : RealImagToComplex
  Scope : Scope  NumInputPorts=3
      settings: YMin=-5~-5~-5  YMax=5~5~5
  Scope1 : Scope  NumInputPorts=3
      settings: YMin=-5~-5~-5  YMax=5~5~5
  Scope2 : Scope  NumInputPorts=5
      settings: YMin=-5~-5~-5~-5~-5  YMax=5~5~5~5~5  SaveName=ScopeData13
  Scope4 : Scope  NumInputPorts=4
      settings: YMin=-5~-5~-5~-5  YMax=5~5~5~5  SaveName=ScopeData5
  Terminator{1..6,8..12} (11 alike) : Terminator
  cnt7bit_ : xbsIndex_r4/Counter  cnt_type=Free Running  cnt_to=Inf  operation=Up  start_count=0  cnt_by_val=1  arith_type=Unsigned  n_bits=7  bin_pt=0  load_pin=off  rst=on  en=on  explicit_period=on  period=1  dbl_ovrd=off  use_behavioral_HDL=off  implementation=Fabric  block_type=counter
  edge_detect : Subsystem  AncestorBlock=casper_library_misc/edge_detect  mask(edge_detect){edge=Rising, polarity=Active High, x_in=[0 0.08 0.08 0.16 0.16 0.24 0.24 0.32 0.32 0.4], y_in=[-1 -1  1  1  1  1  1  1  1  1], x_out=[0.6 0.68 0.68 0.76 0.76 0.84 0.84 0.92 0.92 1], y_out=[-1 -1  1  1 -1 -1 -1 -1 -1 -1]}
      mask prompts: edge "Edge Type"; polarity "Output Polarity"; x_in "Input X Positions"; y_in "Input Y Positions"; x_out "Output X Positions"; y_out "Output Y Positions"
      mask help: Output is active for one-cycle after each edge of the specified type (i.e. rising, falling or both).
      mask init: same as tesd/edge_detect
      settings: AttributesFormatString=|
      | rising edges
      | active high
      mask Help: Output is active for one-cycle after each edge of the specified type (i.e. rising, falling, or both).  Latency is zero.
      mask TypeOptions edge: Rising | Falling | Both
      mask TypeOptions polarity: Active High | Active Low
      mask Display:
      | plot(x_in_num,0.5+y_in_num*0.2);
      | plot(x_out_num,0.5+y_out_num*0.2);
  imtwiddle_ : xbsIndex_r4/ROM  depth=128  initVector=-sin(2*pi*(0:127)/256)  distributed_mem=Block RAM  rst=off  init_reg=0  en=off  latency=1  gui_display_data_type=Fixed-point  arith_type="Signed  (2's comp)"  n_bits=16  bin_pt=15  preci_type=Single  exp_width=8  frac_width=24  dbl_ovrd=off  optimize=Area  use_rpm=on  block_type=sprom
  imtwiddle_1 : xbsIndex_r4/ROM  depth=128  initVector=-sin(2*pi*(128:255)/256)  distributed_mem=Block RAM  rst=off  init_reg=0  en=off  latency=1  gui_display_data_type=Fixed-point  arith_type="Signed  (2's comp)"  n_bits=16  bin_pt=15  preci_type=Single  exp_width=8  frac_width=24  dbl_ovrd=off  optimize=Area  use_rpm=on  block_type=sprom
  retwitddle_ : xbsIndex_r4/ROM  depth=128  initVector=cos(2*pi*(0:127)/256)  distributed_mem=Block RAM  rst=off  init_reg=0  en=off  latency=1  gui_display_data_type=Fixed-point  arith_type="Signed  (2's comp)"  n_bits=16  bin_pt=14  preci_type=Single  exp_width=8  frac_width=24  dbl_ovrd=off  optimize=Area  use_rpm=on  block_type=sprom
  retwitddle_1 : xbsIndex_r4/ROM  depth=128  initVector=cos(2*pi*(128:255)/256)  distributed_mem=Block RAM  rst=off  init_reg=0  en=off  latency=1  gui_display_data_type=Fixed-point  arith_type="Signed  (2's comp)"  n_bits=16  bin_pt=14  preci_type=Single  exp_width=8  frac_width=24  dbl_ovrd=off  optimize=Area  use_rpm=on  block_type=sprom
  uint1_0_1 : xbsIndex_r4/Constant  const=1  gui_display_data_type=Fixed-point  arith_type=Unsigned  n_bits=1  bin_pt=0  preci_type=Single  exp_width=8  frac_width=24  explicit_period=on  period=1  equ=P=C  opselect=C  inp2=PCIN>>17  opr=+  inp1=P  carry=CIN  dbl_ovrd=off  block_type=constant
  OutIm0 : Outport
  dvld : Outport  Port=2
  OutRe0 : Outport  Port=3
  syncout : Outport  Port=4
  OutIm1 : Outport  Port=5
  OutRe1 : Outport  Port=6
  wires:
  Delay10/1 -> Butterfly/7(dvld)
  Gateway Out16/1 -> Scope4/4
  Re1/1 -> Fast Fourier Transform 8.0 1/5, Gateway Out9/1
  Delay3/1 -> Butterfly/4(ReInTw)
  Fast Fourier Transform 8.0 1/5 -> Terminator2/1
  "Fast Fourier Transform 8.0 "/5 -> Delay11/1, Delay10/1, cnt7bit_/2
  Delay9/1 -> Butterfly1/8(syncin)
  retwitddle_1/1 -> Butterfly1/6(TwRe)
  "Fast Fourier Transform 8.0 "/9 -> Terminator11/1
  Delay8/1 -> Butterfly/8(syncin)
  Gateway Out4/1 -> Real-Imag to Complex1/1
  Delay11/1 -> Butterfly1/7(dvld)
  Fast Fourier Transform 8.0 1/7 -> Terminator3/1
  "Fast Fourier Transform 8.0 "/3 -> Delay4/1, Delay/1, Gateway Out/1
  Real-Imag to Complex1/1 -> Complex to Magnitude-Angle1/1
  retwitddle_/1 -> Gateway Out13/1, Butterfly/6(TwRe)
  Delay/1 -> Butterfly/1(ImInOne)
  Butterfly1/1(Imut) -> OutIm1/1
  imtwiddle_1/1 -> Butterfly1/5(TwIm)
  "Fast Fourier Transform 8.0 "/6 -> Delay8/1, Gateway Out16/1, cnt7bit_/1, Gateway Out2/1
  Delay7/1 -> Butterfly1/3(ImInTw)
  Re0/1 -> Gateway Out7/1, "Fast Fourier Transform 8.0 "/5
  Butterfly/4(syncout) -> syncout/1
  "Fast Fourier Transform 8.0 "/7 -> Terminator9/1
  Fast Fourier Transform 8.0 1/10 -> Terminator6/1
  Gateway Out12/1 -> Scope4/1
  Delay4/1 -> Butterfly1/1(ImInOne)
  Butterfly1/2(ReOut) -> OutRe1/1
  "Fast Fourier Transform 8.0 "/2 -> Terminator8/1
  Butterfly/1(Imut) -> OutIm0/1
  Im0/1 -> Gateway Out6/1, "Fast Fourier Transform 8.0 "/4
  Fast Fourier Transform 8.0 1/8 -> Terminator4/1
  Complex to Magnitude-Angle1/1 -> Scope1/1
  syncin/1 -> "Fast Fourier Transform 8.0 "/7, Fast Fourier Transform 8.0 1/7
  "Fast Fourier Transform 8.0 "/10 -> Terminator12/1
  "Fast Fourier Transform 8.0 "/8 -> Terminator10/1
  Gateway Out1/1 -> Real-Imag to Complex/1
  Butterfly/2(ReOut) -> OutRe0/1
  Fast Fourier Transform 8.0 1/3 -> Delay7/1, Delay2/1, Gateway Out3/1
  Gateway Out14/1 -> Scope4/3
  Complex to Magnitude-Angle/1 -> Scope/1
  "Fast Fourier Transform 8.0 "/4 -> Delay5/1, Delay1/1, Gateway Out1/1
  Delay6/1 -> Butterfly1/4(ReInTw)
  Gateway Out2/1 -> Scope/3
  Delay5/1 -> Butterfly1/2(ReInOne)
  cnt7bit_/1 -> retwitddle_1/1, imtwiddle_1/1, Gateway Out14/1, retwitddle_/1, imtwiddle_/1
  imtwiddle_/1 -> Gateway Out12/1, Butterfly/5(TwIm)
  Fast Fourier Transform 8.0 1/2 -> Terminator1/1
  Complex to Magnitude-Angle/2 -> Scope/2
  Delay2/1 -> Butterfly/3(ImInTw)
  Complex to Magnitude-Angle1/2 -> Scope1/2
  Butterfly/3(dvldout) -> dvld/1
  Gateway Out/1 -> Real-Imag to Complex/2
  Delay1/1 -> Butterfly/2(ReInOne)
  Gateway Out5/1 -> Scope1/3
  Gateway Out13/1 -> Scope4/2
  Fast Fourier Transform 8.0 1/1 -> Logical/2
  Real-Imag to Complex/1 -> Complex to Magnitude-Angle/1
  Im1/1 -> Gateway Out8/1, Fast Fourier Transform 8.0 1/4
  Fast Fourier Transform 8.0 1/6 -> Gateway Out5/1, Delay9/1
  Fast Fourier Transform 8.0 1/9 -> Terminator5/1
  Gateway Out3/1 -> Real-Imag to Complex1/2
  Fast Fourier Transform 8.0 1/4 -> Delay3/1, Delay6/1, Gateway Out4/1
  dvldin/1 -> Gateway Out10/1, "Fast Fourier Transform 8.0 "/6, Fast Fourier Transform 8.0 1/6
  rstn/1 -> "Fast Fourier Transform 8.0 "/8, Fast Fourier Transform 8.0 1/8
  Gateway Out6/1 -> Scope2/1
  Gateway Out7/1 -> Scope2/2
  Gateway Out8/1 -> Scope2/3
  Gateway Out9/1 -> Scope2/4
  Gateway Out10/1 -> Scope2/5
  edge_detect/1(out) -> Delay13/1
  Delay12/1 -> edge_detect/1(in)
  "Fast Fourier Transform 8.0 "/1 -> Logical/1
  uint1_0_1/1 -> Fast Fourier Transform 8.0 1/2, "Fast Fourier Transform 8.0 "/2
  Delay13/1 -> Fast Fourier Transform 8.0 1/3, "Fast Fourier Transform 8.0 "/3
  Logical/1 -> Delay12/1
  shift/1 -> Fast Fourier Transform 8.0 1/1, "Fast Fourier Transform 8.0 "/1
